simulink model "Prj_ControleEE_ObsPert2"  (R2016b)
settings: Solver=ode45  StartTime=0.0  StopTime=30  RelTol=1e-6  EnableMultiTasking=on
values from neighbouring files (symbols this model uses):
  L = L'    [PrObsPertContinuoRed.m]    (also in PrPara2nl_PI.m; TestesEE.m; TestesEEcanalI.m; TestesEEobsPert.m)
  Lc = L(4)    [TestesEEcanalI.m]    (also in TestesEEobsPert.m)
  Ls1 = L(4)    [PrObsPertContinuoRed.m]    (also in TestesEEobsPert.m = L(5))
  Ls2 = L(5)    [PrObsPertContinuoRed.m]    (also in TestesEEobsPert.m = L(6))
  Nb = gf.den{1}(1,2)/gf.num{1}(1,2)    [PrObsPertContinuoRed.m]    (also in PrPara2nl_PI.m = gf.den{1}(1,3)/gf.num{1}(1,3); TestesEE.m = gf.den{1}(1,4)/gf.num{1}(1,4); TestesEEcanalI.m = gf.den{1}(1,4)/gf.num{1}(1,4); TestesEEobsPert.m = gf.den{1}(1,4)/gf.num{1}(1,4))
  w0 = .5    (= 0.5)    [PrObsPertContinuoRed.m]    (also in TestesEEobsPert.m)
settings Model: Creator=Adolfo  LastModifiedBy=adolfobs
settings DataIOCC: LimitDataPoints=on  SaveFormat=Array  SignalLoggingSaveFormat=ModelDataLogs
settings OptimizationCC: ExpressionDepthLimit=2147483647  InitFltsAndDblsToZero=on  LifeSpan=inf
settings DebuggingCC: SaveWithParameterizedLinksMsg=none  UnderspecifiedInitializationDetection=Classic  MergeDetectMultiDrivingBlocksExec=none  SignalResolutionControl=TryResolveAllWithWarning  SolverPrmCheckMsg=warning  MultiTaskDSMMsg=warning  MultiTaskCondExecSysMsg=none  FcnCallInpInsideContextMsg=warning  StateNameClashWarn=warning  SFUnexpectedBacktrackingDiag=warning  SFNoUnconditionalDefaultTransitionDiag=warning  SFExecutionAtInitializationDiag=none
settings HardwareCC: ProdBitPerPointer=32  ProdBitPerSizeT=32  ProdBitPerPtrDiffT=32  ProdLargestAtomicFloat=None  ProdIntDivRoundTo=Undefined  ProdEndianess=Unspecified  ProdWordSize=32  ProdHWDeviceType=32-bit Generic
settings ModelReferenceCC: PropagateSignalLabelsOutOfModel=off
settings GRTTargetCC: TargetFcnLib=ansi_tfl_tmw.mat  TargetLangStandard=C89/C90 (ANSI)  GeneratePreprocessorConditionals=Disable all  CombineOutputUpdateFcns=off  GRTInterface=on
settings ConfigComp: CovMetricSettings=dw  CovHtmlReporting=on  CovSaveCumulativeToWorkspaceVar=on  CovSaveSingleToWorkspaceVar=on  CovExternalEMLEnable=off  CovSFcnEnable=off

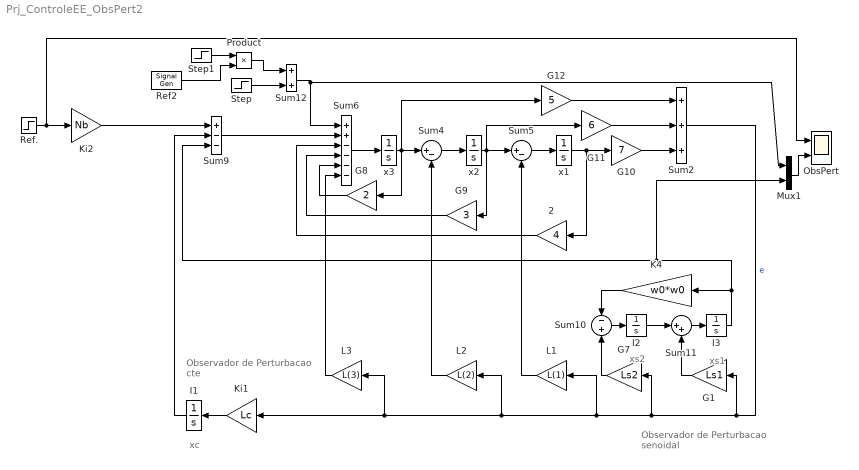
== system Prj_ControleEE_ObsPert2 ==
  note: xc
  note: xs1
  note: xs2
  note: Observador de
      | Perturbacao cte
  note: Observador de
      | Perturbacao senoidal
  2 : Gain  Gain=4
  G1 : Gain  Gain=Ls1  SaturateOnIntegerOverflow=on  OutDataTypeStr=Inherit: Same as input  ParamDataTypeStr=Inherit: Same as input
  G10 : Gain  Gain=7
  G11 : Gain  Gain=6
  G12 : Gain  Gain=5
  G7 : Gain  Gain=Ls2  SaturateOnIntegerOverflow=on  OutDataTypeStr=Inherit: Same as input  ParamDataTypeStr=Inherit: Same as input
  G8 : Gain  Gain=2
  G9 : Gain  Gain=3
  I1 : Integrator
  I2 : Integrator
  I3 : Integrator
  K4 : Gain  Gain=w0*w0  SaturateOnIntegerOverflow=on  OutDataTypeStr=Inherit: Same as input  ParamDataTypeStr=Inherit: Same as input
  Ki1 : Gain  Gain=Lc
  Ki2 : Gain  Gain=Nb
  L1 : Gain  Gain=L(1)
  L2 : Gain  Gain=L(2)
  L3 : Gain  Gain=L(3)
  Mux1 : Mux  Inputs=2
  ObsPert : Scope  NumInputPorts=2
  Product : Product
  Ref. : Step  Time=0  SampleTime=0
  Ref2 : SignalGenerator  Amplitude=20  Frequency=w0  Units=rad/sec
  Step : Step  Time=3  SampleTime=0
  Step1 : Step  Time=2*pi/w0  SampleTime=0
  Sum10 : Sum  Inputs=-+  SaturateOnIntegerOverflow=on  InputSameDT=on  OutDataTypeStr=Inherit: Same as first input
  Sum11 : Sum  Inputs=|++  SaturateOnIntegerOverflow=on  InputSameDT=on  OutDataTypeStr=Inherit: Same as first input
  Sum12 : Sum
  Sum2 : Sum  Inputs=+++
  Sum4 : Sum  Inputs=|+-
  Sum5 : Sum  Inputs=|+-
  Sum6 : Sum  Inputs=++----
  Sum9 : Sum  Inputs=+--
  x1 : Integrator
  x2 : Integrator
  x3 : Integrator
  wires:
  Ref./1 -> ObsPert/1, Ki2/1
  Ki2/1 -> Sum9/1
  Sum10/1 -> I2/1
  Sum11/1 -> I3/1
  K4/1 -> Sum10/1
  I2/1 -> Sum11/1
  G1/1 -> Sum11/2
  G7/1 -> Sum10/2
  Sum9/1 -> Sum6/2
  Mux1/1 -> ObsPert/2
  Step/1 -> Sum12/2
  Sum12/1 -> Sum6/1, Mux1/1
  I3/1 -> K4/1, Mux1/2, Sum9/3
  Step1/1 -> Product/1
  Ref2/1 -> Product/2
  Product/1 -> Sum12/1
  Ki1/1 -> I1/1
  I1/1 -> Sum9/2
  Sum6/1 -> x3/1
  G8/1 -> Sum6/5
  G9/1 -> Sum6/4
  x1/1 -> G10/1, 2/1
  2/1 -> Sum6/3
  G10/1 -> Sum2/3
  G11/1 -> Sum2/2
  G12/1 -> Sum2/1
  x3/1 -> Sum4/1, G12/1, G8/1
  Sum2/1 -> L1/1, L2/1, L3/1, Ki1/1, G7/1, G1/1  "e"
  Sum4/1 -> x2/1
  x2/1 -> Sum5/1, G11/1, G9/1
  Sum5/1 -> x1/1
  L1/1 -> Sum5/2
  L2/1 -> Sum4/2
  L3/1 -> Sum6/6
